simulink model "test"  (Simulink 7.7)
settings: Solver=FixedStepDiscrete  StartTime=0.0  StopTime=1000  FixedStep=0.01  RelTol=1e-3
PreLoadFcn:
  | robotName = 'icubGazeboSim';
  | localName = 'SimulinkiCubGazeboSim';
InitFcn:
  | robotName = 'icubGazeboSim';
  | localName = 'SimulinkiCubGazeboSim';
libraries: WBCLibrary x2
settings Model: Creator=iron  LastModifiedBy=iron

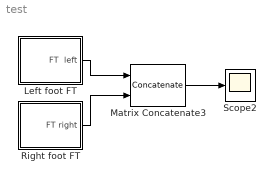
== system test ==
  Left foot FT : Subsystem
  Matrix Concatenate3 : Concatenate  Mode=Multidimensional array
  Right foot FT : Subsystem
  Scope2 : Scope
      settings: TimeRange=1000
  wires:
  Left foot FT/1(FT  left) -> Matrix Concatenate3/1
  Right foot FT/1(FT right) -> Matrix Concatenate3/2
  Matrix Concatenate3/1 -> Scope2/1

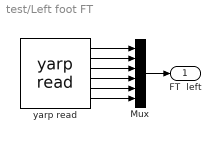
== system test/Left foot FT ==
  Mux : Mux  Inputs=6
  yarp read : WBCLibrary/Utilities/yarp read  from=['/' robotName '/left_foot/analog:o']  to='/left_foot/FT'  num=6
  FT  left : Outport
  wires:
  yarp read/1 -> Mux/1
  yarp read/2 -> Mux/2
  yarp read/3 -> Mux/3
  yarp read/4 -> Mux/4
  yarp read/5 -> Mux/5
  yarp read/6 -> Mux/6
  Mux/1 -> FT  left/1

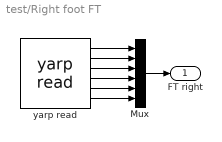
== system test/Right foot FT ==
  Mux : Mux  Inputs=6
  yarp read : WBCLibrary/Utilities/yarp read  from=['/' robotName '/right_foot/analog:o']  to='/right_foot/FT'  num=6
  FT right : Outport
  wires:
  yarp read/1 -> Mux/1
  yarp read/2 -> Mux/2
  yarp read/3 -> Mux/3
  yarp read/4 -> Mux/4
  yarp read/5 -> Mux/5
  yarp read/6 -> Mux/6
  Mux/1 -> FT right/1
